simulink model "feedback_control_tuning"  (R2018a)
settings: Solver=FixedStepAuto  StartTime=0.0  StopTime=inf  FixedStep=0.01  RelTol=1e-3  EnableMultiTasking=on
undefined symbols (not defined in the file): CR, LF, serial
libraries: instrumentlib x3, simulink x2
settings Model: Creator=Hp2  LastModifiedBy=Hp2
settings SolverCC: PositivePriorityOrder=on
settings DataIOCC: LimitDataPoints=on  SaveFormat=Array
settings OptimizationCC: LifeSpan=inf
settings DebuggingCC: UnderspecifiedInitializationDetection=Classic  MergeDetectMultiDrivingBlocksExec=none  SolverPrmCheckMsg=warning  StateNameClashWarn=warning  SFUnexpectedBacktrackingDiag=warning  SFNoUnconditionalDefaultTransitionDiag=warning  SFExecutionAtInitializationDiag=none
settings HardwareCC: ProdBitPerPointer=32  ProdBitPerSizeT=32  ProdBitPerPtrDiffT=32  ProdLargestAtomicFloat=None  ProdIntDivRoundTo=Undefined  ProdEndianess=Unspecified  ProdWordSize=32  ProdHWDeviceType=32-bit Generic
settings ModelReferenceCC: PropagateSignalLabelsOutOfModel=off
settings CodeAppCC: StateflowObjectComments=on
settings GRTTargetCC: TargetLangStandard=C89/C90 (ANSI)  GeneratePreprocessorConditionals=Disable all
settings ConfigComp: CovMetricSettings=dw  CovHtmlReporting=on  CovSaveCumulativeToWorkspaceVar=on  CovSaveSingleToWorkspaceVar=on  CovExternalEMLEnable=off

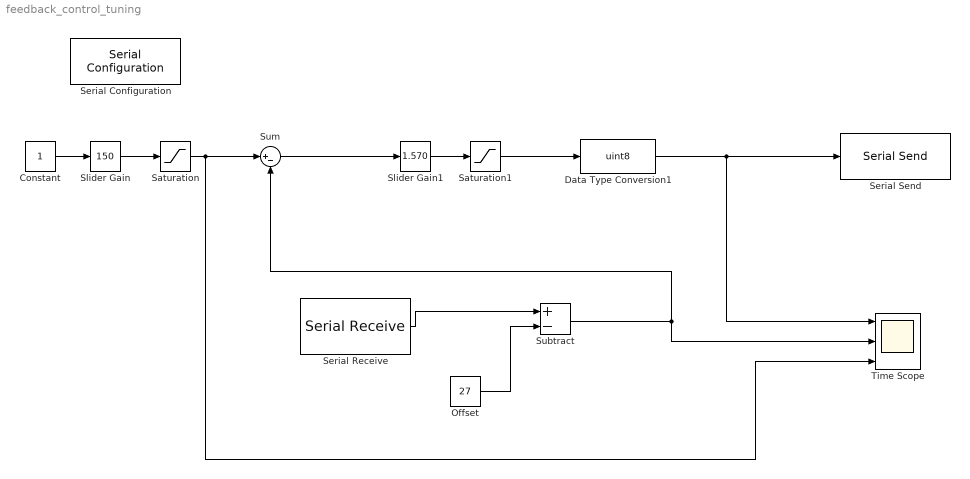
== system feedback_control_tuning ==
  Constant : Constant  OutDataTypeStr=uint16  SampleTime=-1
  Data Type Conversion1 : DataTypeConversion  OutDataTypeStr=uint8
  Offset : Constant  Value=27  OutDataTypeStr=uint16  SampleTime=0.01
  Saturation : Saturate  UpperLimit=1000  LowerLimit=1
  Saturation1 : Saturate  UpperLimit=255  LowerLimit=0
  Serial Configuration : instrumentlib/Serial Configuration  Priority=-200000  ComPortMenu=<Please select a port...>  ComPort=COM6  ObjConstructor=serial('COM6');  BaudRate=19200  DataBits=8  Parity=none  StopBits=1  FlowControl=none  Timeout=10  ByteOrder=LittleEndian
  Serial Receive : instrumentlib/Serial Receive  ComPortMenu=COM6  ComPort=COM6  ObjConstructor=serial('COM6');  Terminator=CR/LF ('\r\n')  DataSize=1  DataType=uint16  EnableBlockingMode=on  ActionDataUnavailable=Output last received value  CustomValue=0  SampleTime=-1
  Serial Send : instrumentlib/Serial Send  ComPortMenu=<Please select a port...>  ComPort=COM6  ObjConstructor=serial('COM6');  Terminator=<none>  EnableBlockingMode=off
  Slider Gain : simulink/Math Operations/Slider Gain  gain=150  low=1  high=1000
  Slider Gain1 : simulink/Math Operations/Slider Gain  gain=1.570  low=1  high=20
  Subtract : Sum  Inputs=+-  OutDataTypeStr=int16
  Sum : Sum  Inputs=|+-  AccumDataTypeStr=uint16  OutDataTypeStr=int16
  Time Scope : Scope  NumInputPorts=3
  wires:
  Saturation/1 -> Time Scope/3, Sum/1
  Constant/1 -> Slider Gain/1
  Slider Gain/1 -> Saturation/1
  Serial Receive/1 -> Subtract/1
  Subtract/1 -> Sum/2, Time Scope/2
  Offset/1 -> Subtract/2
  Data Type Conversion1/1 -> Time Scope/1, Serial Send/1
  Slider Gain1/1 -> Saturation1/1
  Saturation1/1 -> Data Type Conversion1/1
  Sum/1 -> Slider Gain1/1
